simulink model "chap02_03_43_mdl"  (R2013b)
settings: Solver=ode45  StartTime=0.0  StopTime=20  MaxStep=0.01  RelTol=1e-3
settings Model: Creator=Administrator  LastModifiedBy=sunzx.fnst

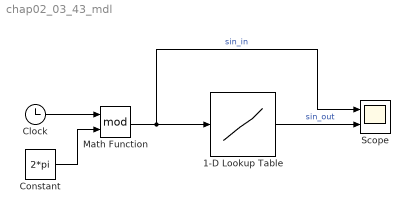
== system chap02_03_43_mdl ==
  1-D Lookup Table : Lookup_n-D  NumberOfTableDimensions=1  BreakpointsForDimension1=linspace(0,2*pi,256)  Table=sin(linspace(0,2*pi,256))  InternalRulePriority=Speed  RndMeth=Simplest  InputSameDT=on
  Clock : Clock
  Constant : Constant  Value=2*pi
  Math Function : Math  Operator=mod  SaturateOnIntegerOverflow=on
  Scope : Scope  NumInputPorts=2
      settings: YMin=-5~-5  YMax=5~5
  wires:
  Clock/1 -> Math Function/1
  Constant/1 -> Math Function/2
  Math Function/1 -> Scope/1, 1-D Lookup Table/1  "sin_in"
  1-D Lookup Table/1 -> Scope/2  "sin_out"
